simulink model "Lat_Rate_Damper"  (R2024b)
settings: Solver=VariableStepAuto  StartTime=0.0  StopTime=200  RelTol=1e-3
undefined symbols (not defined in the file or in its folder): Ki_a, Ki_b, Kp_a, Kp_b
libraries: slpidlib x2
settings Model: Creator=GH-X-ST  LastModifiedBy=GH-X-ST

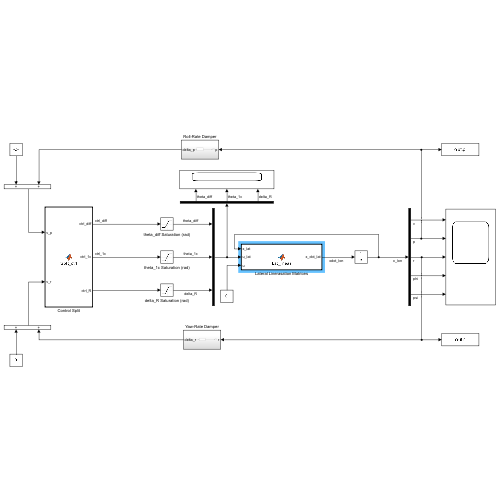
[thumbnail: Simulink's stored preview of the top-level diagram]
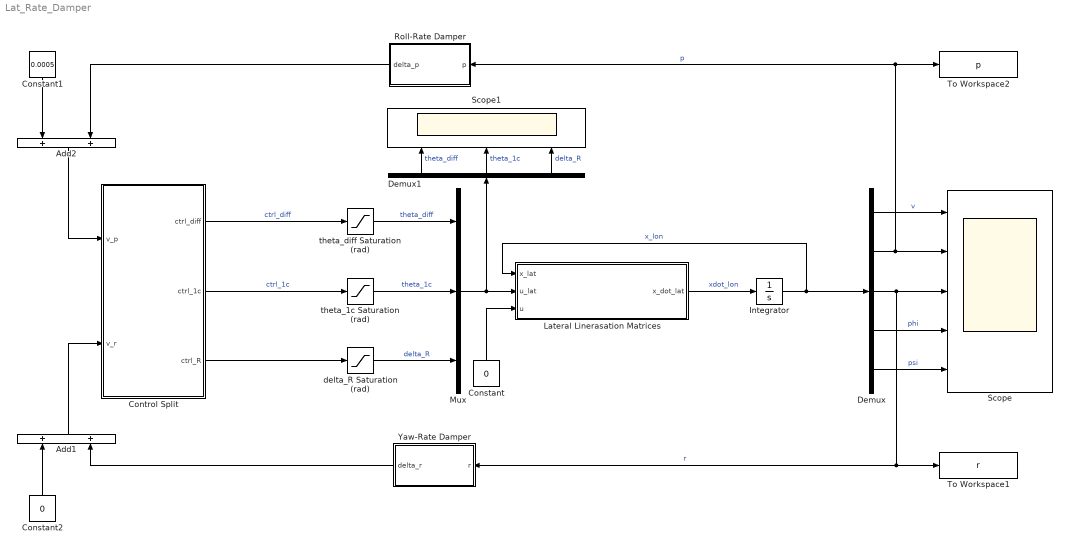
== system Lat_Rate_Damper ==
  Add1 : Sum
  Add2 : Sum
  Constant : Constant  Value=0
  Constant1 : Constant  Value=0.0005
  Constant2 : Constant  Value=0
  Control Split : MATLAB Function  TreatAsAtomicUnit=on
  Demux : Demux  Outputs=5
  Demux1 : Demux  Outputs=3
  Integrator : Integrator  InitialCondition=[0;0;0;0;0]
  Lateral Linerasation Matrices : MATLAB Function  TreatAsAtomicUnit=on
  Mux : Mux  Inputs=3
  Roll-Rate Damper : Subsystem
  Scope : Scope  NumInputPorts=5
  Scope1 : Scope  NumInputPorts=3
  To Workspace1 : ToWorkspace  VariableName=r  SaveFormat=Timeseries  SampleTime=-1
  To Workspace2 : ToWorkspace  VariableName=p  SaveFormat=Timeseries  SampleTime=-1
  Yaw-Rate Damper : Subsystem
  delta_R Saturation (rad) : Saturate  UpperLimit=deg2rad(11)  LowerLimit=deg2rad(-11)
  theta_1c Saturation (rad) : Saturate  UpperLimit=deg2rad(3)  LowerLimit=deg2rad(-3)
  theta_diff Saturation (rad) : Saturate  UpperLimit=deg2rad(5)  LowerLimit=deg2rad(-5)
  wires:
  Lateral Linerasation Matrices/1(x_dot_lat) -> Integrator/1  "xdot_lon"
  Integrator/1 -> Lateral Linerasation Matrices/1(x_lat), Demux/1  "x_lon"
  Demux/1 -> Scope/1  "v"
  Demux/2 -> Roll-Rate Damper/1(p), To Workspace2/1, Scope/2  "p"
  Demux/3 -> Scope/3, To Workspace1/1, Yaw-Rate Damper/1(r)  "r"
  Demux/4 -> Scope/4  "phi"
  delta_R Saturation (rad)/1 -> Mux/3  "delta_R"
  Mux/1 -> Demux1/1, Lateral Linerasation Matrices/2(u_lat)
  Demux1/3 -> Scope1/3  "delta_R"
  Demux1/2 -> Scope1/2  "theta_1c"
  Demux1/1 -> Scope1/1  "theta_diff"
  Demux/5 -> Scope/5  "psi"
  theta_diff Saturation (rad)/1 -> Mux/1  "theta_diff"
  theta_1c Saturation (rad)/1 -> Mux/2  "theta_1c"
  Constant1/1 -> Add2/1
  Roll-Rate Damper/1(delta_p) -> Add2/2
  Add2/1 -> Control Split/1(v_p)
  Constant/1 -> Lateral Linerasation Matrices/3(u)
  Control Split/1(ctrl_diff) -> theta_diff Saturation (rad)/1  "ctrl_diff"
  Control Split/2(ctrl_1c) -> theta_1c Saturation (rad)/1  "ctrl_1c"
  Add1/1 -> Control Split/2(v_r)
  Yaw-Rate Damper/1(delta_r) -> Add1/2
  Constant2/1 -> Add1/1
  Control Split/3(ctrl_R) -> delta_R Saturation (rad)/1

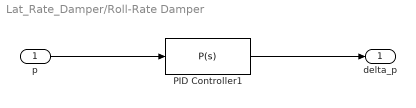
== system Lat_Rate_Damper/Roll-Rate Damper ==
  p : Inport
  PID Controller1 : slpidlib/PID Controller  Controller=P  Form=Parallel  TimeDomain=Continuous-time  UseExternalTs=off  SampleTime=-1  IntegratorMethod=Forward Euler  FilterMethod=Forward Euler  ControllerParametersSource=internal  P=Kp_a  I=Ki_a  UseKiTs=off  D=0.005  UseExternalDerivativeSource=on  N=100  UseFilter=on  TunerSelectOption=Transfer Function Based (PID Tuner App)  InitialConditionSource=internal  InitialConditionForIntegrator=0  InitialConditionForFilter=0  DifferentiatorICPrevScaledInput=0  ExternalReset=none  TrackingMode=off  Kt=1  LimitOutput=on  SatLimitsSource=internal  UpperSaturationLimit=1  LowerSaturationLimit=-1  LinearizeAsGain=on  AntiWindupMode=none  Kb=1  LimitIntegrator=off  UpperIntegratorSaturationLimit=inf  LowerIntegratorSaturationLimit=-inf  POutMin=[]  POutMax=[]  IOutMin=[]  IOutMax=[]  DOutMin=[]  DOutMax=[]  NOutMin=[]  NOutMax=[]  SumOutMin=[]  SumOutMax=[]  SaturationOutMin=[]  SaturationOutMax=[]  PParamMin=[]  PParamMax=[]  IParamMin=[]  IParamMax=[]  DParamMin=[]  DParamMax=[]  NParamMin=[]  NParamMax=[]  KbParamMin=[]  KbParamMax=[]  KtParamMin=[]  KtParamMax=[]  KbOutMin=[]  KbOutMax=[]  KtOutMin=[]  KtOutMax=[]  IntegratorOutMin=[]  IntegratorOutMax=[]  FilterOutMin=[]  FilterOutMax=[]  SumI1OutMin=[]  SumI1OutMax=[]  SumI2OutMin=[]  SumI2OutMax=[]  SumI3OutMin=[]  SumI3OutMax=[]  SumI4OutMin=[]  SumI4OutMax=[]  SumDOutMin=[]  SumDOutMax=[]  DifferentiatorOutMin=[]  DifferentiatorOutMax=[]  FilterDiffOutCoefMin=[]  FilterDiffOutCoefMax=[]  ReciprocalOutMin=[]  ReciprocalOutMax=[]  SumDenOutMin=[]  SumDenOutMax=[]  SumNumOutMin=[]  SumNumOutMax=[]  DivideOutMin=[]  DivideOutMax=[]  UdiffTsProdOutMin=[]  UdiffTsProdOutMax=[]  NTsProdOutMin=[]  NTsProdOutMax=[]  UintegralTsProdOutMin=[]  UintegralTsProdOutMax=[]  UngainTsProdOutMin=[]  UngainTsProdOutMax=[]  ClampingZeroOutDataTypeStr=Inherit: Inherit via back propagation  ClampingZeroOutMin=[]  ClampingZeroOutMax=[]  FilterDenConstantOutDataTypeStr=Inherit: Inherit via back propagation  FilterDenConstantOutMin=[]  FilterDenConstantOutMax=[]  PCopyOutDataTypeStr=Inherit: Inherit via back propagation  PCopyOutMin=[]  PCopyOutMax=[]  NCopyOutDataTypeStr=Inherit: Inherit via back propagation  NCopyOutMin=[]  NCopyOutMax=[]  IntegratorContinuousStateAttributes=''  IntegratorStateMustResolveToSignalObject=off  IntegratorRTWStateStorageClass=Auto  FilterContinuousStateAttributes=''  FilterStateMustResolveToSignalObject=off  FilterRTWStateStorageClass=Auto  ParallelPVariant=InternalParameters  IdealPVariant=Disabled  IVariant=Disabled  DVariant=Disabled  IntegratorVariant=Disabled  SatVariant=Enabled  AWVariant=Disabled  PCopyVariant=Disabled  TRVariant=Disabled  FdbkBlocksVariant=Forward  IdealPFdbkVariant=Disabled  SatFdbkVariant=Disabled  DerivativeFilterVariant=Disabled  NVariant=Passthrough  NCopyVariant=Disabled_SignalSpec  FilterICVariant=Disabled  IntegratorICVariant=Disabled  ExternalResetVariant=Disabled  TRSumVariant=Passthrough  SumFdbkVariant=Disabled  SumVariant=Passthrough_P  TsampFilterVariant=InternalTs  TsampNgainVariant=Passthrough  TsampIntegralVariant=Disabled_SignalSpec  ExternalSaturationOutDataTypeStr=Inherit: Same as second input  DerivativeSourceVariant=Disabled  PreIntVariant=InternalPreInt
  delta_p : Outport
  wires:
  PID Controller1/1 -> delta_p/1
  p/1 -> PID Controller1/1

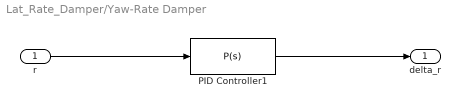
== system Lat_Rate_Damper/Yaw-Rate Damper ==
  r : Inport
  PID Controller1 : slpidlib/PID Controller  Controller=P  Form=Parallel  TimeDomain=Continuous-time  UseExternalTs=off  SampleTime=-1  IntegratorMethod=Forward Euler  FilterMethod=Forward Euler  ControllerParametersSource=internal  P=Kp_b  I=Ki_b  UseKiTs=off  D=0.005  UseExternalDerivativeSource=on  N=100  UseFilter=on  TunerSelectOption=Transfer Function Based (PID Tuner App)  InitialConditionSource=internal  InitialConditionForIntegrator=0  InitialConditionForFilter=0  DifferentiatorICPrevScaledInput=0  ExternalReset=none  TrackingMode=off  Kt=1  LimitOutput=on  SatLimitsSource=internal  UpperSaturationLimit=1  LowerSaturationLimit=-1  LinearizeAsGain=on  AntiWindupMode=none  Kb=1  LimitIntegrator=off  UpperIntegratorSaturationLimit=inf  LowerIntegratorSaturationLimit=-inf  POutMin=[]  POutMax=[]  IOutMin=[]  IOutMax=[]  DOutMin=[]  DOutMax=[]  NOutMin=[]  NOutMax=[]  SumOutMin=[]  SumOutMax=[]  SaturationOutMin=[]  SaturationOutMax=[]  PParamMin=[]  PParamMax=[]  IParamMin=[]  IParamMax=[]  DParamMin=[]  DParamMax=[]  NParamMin=[]  NParamMax=[]  KbParamMin=[]  KbParamMax=[]  KtParamMin=[]  KtParamMax=[]  KbOutMin=[]  KbOutMax=[]  KtOutMin=[]  KtOutMax=[]  IntegratorOutMin=[]  IntegratorOutMax=[]  FilterOutMin=[]  FilterOutMax=[]  SumI1OutMin=[]  SumI1OutMax=[]  SumI2OutMin=[]  SumI2OutMax=[]  SumI3OutMin=[]  SumI3OutMax=[]  SumI4OutMin=[]  SumI4OutMax=[]  SumDOutMin=[]  SumDOutMax=[]  DifferentiatorOutMin=[]  DifferentiatorOutMax=[]  FilterDiffOutCoefMin=[]  FilterDiffOutCoefMax=[]  ReciprocalOutMin=[]  ReciprocalOutMax=[]  SumDenOutMin=[]  SumDenOutMax=[]  SumNumOutMin=[]  SumNumOutMax=[]  DivideOutMin=[]  DivideOutMax=[]  UdiffTsProdOutMin=[]  UdiffTsProdOutMax=[]  NTsProdOutMin=[]  NTsProdOutMax=[]  UintegralTsProdOutMin=[]  UintegralTsProdOutMax=[]  UngainTsProdOutMin=[]  UngainTsProdOutMax=[]  ClampingZeroOutDataTypeStr=Inherit: Inherit via back propagation  ClampingZeroOutMin=[]  ClampingZeroOutMax=[]  FilterDenConstantOutDataTypeStr=Inherit: Inherit via back propagation  FilterDenConstantOutMin=[]  FilterDenConstantOutMax=[]  PCopyOutDataTypeStr=Inherit: Inherit via back propagation  PCopyOutMin=[]  PCopyOutMax=[]  NCopyOutDataTypeStr=Inherit: Inherit via back propagation  NCopyOutMin=[]  NCopyOutMax=[]  IntegratorContinuousStateAttributes=''  IntegratorStateMustResolveToSignalObject=off  IntegratorRTWStateStorageClass=Auto  FilterContinuousStateAttributes=''  FilterStateMustResolveToSignalObject=off  FilterRTWStateStorageClass=Auto  ParallelPVariant=InternalParameters  IdealPVariant=Disabled  IVariant=Disabled  DVariant=Disabled  IntegratorVariant=Disabled  SatVariant=Enabled  AWVariant=Disabled  PCopyVariant=Disabled  TRVariant=Disabled  FdbkBlocksVariant=Forward  IdealPFdbkVariant=Disabled  SatFdbkVariant=Disabled  DerivativeFilterVariant=Disabled  NVariant=Passthrough  NCopyVariant=Disabled_SignalSpec  FilterICVariant=Disabled  IntegratorICVariant=Disabled  ExternalResetVariant=Disabled  TRSumVariant=Passthrough  SumFdbkVariant=Disabled  SumVariant=Passthrough_P  TsampFilterVariant=InternalTs  TsampNgainVariant=Passthrough  TsampIntegralVariant=Disabled_SignalSpec  ExternalSaturationOutDataTypeStr=Inherit: Same as second input  DerivativeSourceVariant=Disabled  PreIntVariant=InternalPreInt
  delta_r : Outport
  wires:
  PID Controller1/1 -> delta_r/1
  r/1 -> PID Controller1/1

== matlab function Lat_Rate_Damper/Lateral Linerasation Matrices ==
  data: x_lat input; u_lat input; u input; x_dot_lat output
function x_dot_lat = Lat_linear(x_lat, u_lat, u)
% Author:
%   Hanchen Li (hl3422@ic.ac.uk)
%
% Inputs:
%   x_lat     - [v, p, r, phi, psi]
%   v         - Lateral velocity (m/s)
%   p         - Roll rate (rad/s)
%   r         - Yaw rate (rad/s)
%   phi       - Euler roll angle (rad)
%   psi       - Euler yaw angle (rad)
%
%   u_lat      - [theta_diff, theta_1c, delta_R]
%   theta_diff - Rotor collective difference (rad)
%   theta_1c   - Lateral cyclic (rad)
%   delta_R    - Rudder deflection (rad)
%
%   u         - Forward velocity (m/s)
%
% Outputs:
%   x_dot_lat

A_lat = ...
[-0.0270930792327373	-0.499103864580706	-10.0100000000000	9.79657549425923	0;
0.101333813739032	-44.9802037301025	0	0	0;
0.0312667638212951	-17.2233534731576	0	0	0;
0	1	0.0450899242286570	0	0;
0	0	1.00100375056752	0	0];

B_lat = ...
[1.91673446434639	2.90610088393772	-0.301307431814120;
-69.8736584213303	441.417104012504	-0.239321802736061;
-26.8554762228028	169.023890718703	-0.166811869505905;
0	0	0;
0	0	0];

x_dot_lat = A_lat * x_lat + B_lat * u_lat;

end

== matlab function Lat_Rate_Damper/Control Split ==
  data: ctrl_diff output; ctrl_1c output; v_p input; v_r input; ctrl_R output
function [ctrl_diff, ctrl_1c, ctrl_R] = Split_ctrl(v_p, v_r)
% Author:
%   Hanchen Li (hl3422@ic.ac.uk)
%
% Inputs:
%   v_p       - desire roll rate
%   v_r       - desire yaw rate
%
% Outputs:
%   u_ctrl     - [theta_diff, theta_1c, delta_R]

B_lat = ...
[1.91673446434639	2.90610088393772	-0.301307431814120;
-69.8736584213303	441.417104012504	-0.239321802736061;
-26.8554762228028	169.023890718703	-0.166811869505905;
0	0	0;
0	0	0];

B_LN = B_lat([2,3], :);

lambda = 1e-4;
u_ctrl = (B_LN' * B_LN + lambda * eye(3)) \ (B_LN' * [v_p; v_r]);

cond_B = cond(B_LN);
disp(['cond(B_LN) = ', num2str(cond_B)]);

ctrl_diff = u_ctrl(1);

ctrl_1c = u_ctrl(2);

ctrl_R = u_ctrl(3);

end
